simulink model "force"  (R2017a)
settings: Solver=VariableStepAuto  StartTime=0.0  StopTime=10.0  RelTol=1e-3
values from neighbouring files (symbols this model uses):
  F_max = 0.45*[ 1850;2370;2190;400;1000;5200;1600;3600;1100]    [total_force.m]
settings Model: Creator=Nathaniel  LastModifiedBy=Nathaniel

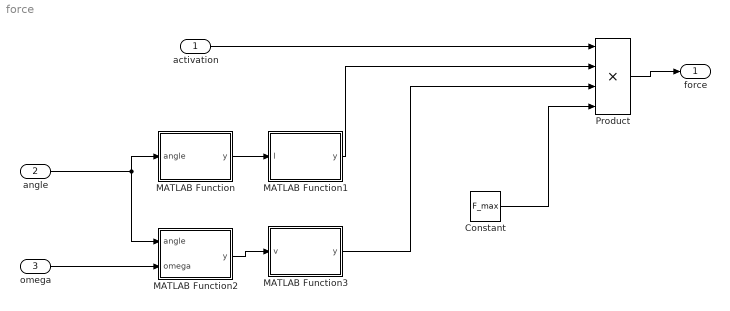
== system force ==
  activation : Inport
  angle : Inport  Port=2
  omega : Inport  Port=3
  Constant : Constant  Value=F_max
  MATLAB Function : MATLAB Function  TreatAsAtomicUnit=on
  MATLAB Function1 : MATLAB Function  TreatAsAtomicUnit=on
  MATLAB Function2 : MATLAB Function  TreatAsAtomicUnit=on
  MATLAB Function3 : MATLAB Function  TreatAsAtomicUnit=on
  Product : Product  Inputs=4
  force : Outport
  wires:
  activation/1 -> Product/1
  MATLAB Function/1(y) -> MATLAB Function1/1(l)
  MATLAB Function1/1(y) -> Product/2
  angle/1 -> MATLAB Function/1(angle), MATLAB Function2/1(angle)
  MATLAB Function2/1(y) -> MATLAB Function3/1(v)
  MATLAB Function3/1(y) -> Product/3
  omega/1 -> MATLAB Function2/2(omega)
  Constant/1 -> Product/4
  Product/1 -> force/1

== matlab function force/MATLAB Function1 ==
  data: l input; y output
function y = fcn(l)

y = force_length(l);

== matlab function force/MATLAB Function ==
  data: angle input; y output
function y = fcn(angle)

y = normL(angle);

== matlab function force/MATLAB Function2 ==
  data: angle input; y output; omega input
function y = fcn(angle,omega)

y = normV(angle,omega);

== matlab function force/MATLAB Function3 ==
  data: v input; y output
function y = fcn(v)

y = force_velocity(v);
